simulink model "myModel"  (R2024b)
settings: Solver=ode15s  StartTime=0.0  StopTime=10.0  RelTol=1e-3
undefined symbols (not defined in the file): setpoint
settings Model: Creator=rodri  LastModifiedBy=rodri

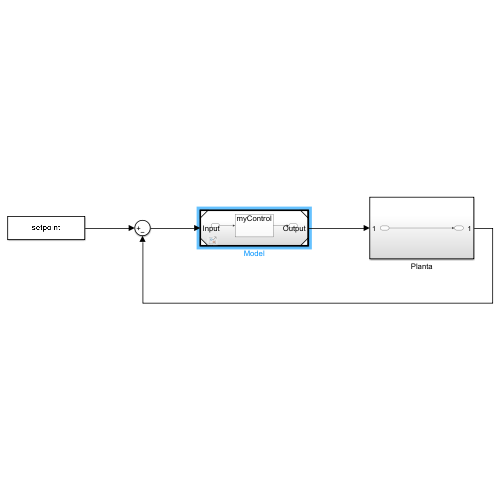
[thumbnail: Simulink's stored preview of the top-level diagram]
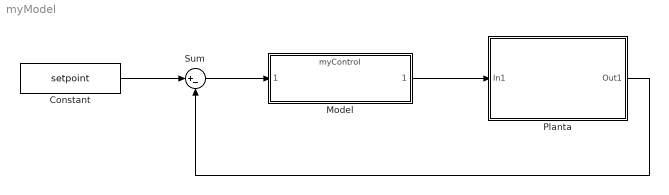
== system myModel ==
  Constant : Constant  Value=setpoint
  Model : ModelReference  ModelNameDialog=myControl.slx  SimulationMode=Normal  ModelReferenceVersion=1.3
  Planta : Subsystem
  Sum : Sum  Inputs=|+-
  wires:
  Sum/1 -> Model/1
  Model/1 -> Planta/1(In1)
  Planta/1(Out1) -> Sum/2
  Constant/1 -> Sum/1

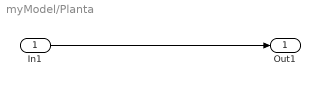
== system myModel/Planta ==
  In1 : Inport
  Out1 : Outport
  wires:
  In1/1 -> Out1/1
